simulink model "GPCA_CONFIGNoActions"  (Simulink 9.0)
settings: Solver=FixedStepDiscrete  StartTime=0.0  StopTime=10.0  RelTol=1e-3  EnableMultiTasking=on
settings Model: SuppressorTable=22 serialization::archive 11 0 6 0 0 0 0 0  Creator=bourbouh  LastModifiedBy=ktrinh
settings DataIOCC: SaveFormat=Dataset
settings DebuggingCC: UnderspecifiedInitializationDetection=Simplified  MergeDetectMultiDrivingBlocksExec=error
settings HardwareCC: ProdBitPerPointer=64  ProdBitPerSizeT=64  ProdBitPerPtrDiffT=64  ProdLargestAtomicFloat=Float  ProdIntDivRoundTo=Zero  ProdEndianess=LittleEndian  ProdWordSize=64  ProdHWDeviceType=Intel->x86-64 (Windows64)
settings ModelReferenceCC: PropagateSignalLabelsOutOfModel=on
settings GRTTargetCC: GeneratePreprocessorConditionals=Disable all

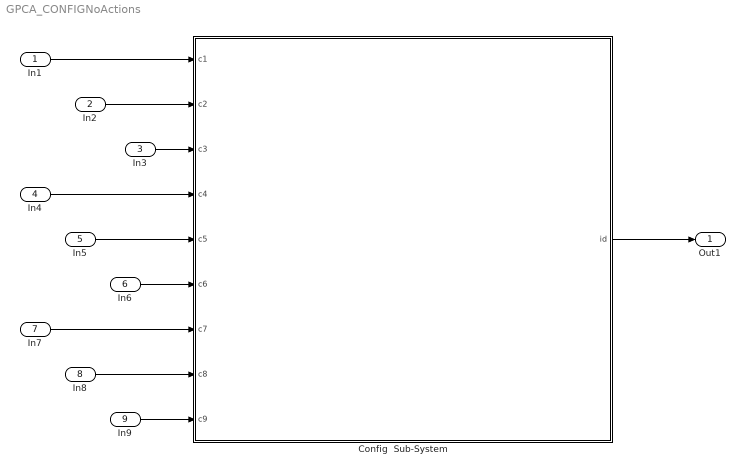
== system GPCA_CONFIGNoActions ==
  In1 : Inport  OutDataTypeStr=boolean
  In2 : Inport  Port=2  OutDataTypeStr=boolean
  In3 : Inport  Port=3  OutDataTypeStr=boolean
  In4 : Inport  Port=4  OutDataTypeStr=boolean
  In5 : Inport  Port=5  OutDataTypeStr=boolean
  In6 : Inport  Port=6  OutDataTypeStr=boolean
  In7 : Inport  Port=7  OutDataTypeStr=boolean
  In8 : Inport  Port=8  OutDataTypeStr=boolean
  In9 : Inport  Port=9  OutDataTypeStr=boolean
  Config  Sub-System : Stateflow chart  TreatAsAtomicUnit=on
  Out1 : Outport
  wires:
  Config  Sub-System/1(id) -> Out1/1
  In1/1 -> Config  Sub-System/1(c1)
  In9/1 -> Config  Sub-System/9(c9)
  In8/1 -> Config  Sub-System/8(c8)
  In7/1 -> Config  Sub-System/7(c7)
  In6/1 -> Config  Sub-System/6(c6)
  In5/1 -> Config  Sub-System/5(c5)
  In4/1 -> Config  Sub-System/4(c4)
  In3/1 -> Config  Sub-System/3(c3)
  In2/1 -> Config  Sub-System/2(c2)

== stateflow chart Config  Sub-System ==
  state Configuration
    en: id=2
    state Prescription_Config
      entry: id=22;
      state Patient_Drug_info
        entry: id=221;
        state GetParam
          entry: id = 222;
        state DisplayParam
          entry: id=222;
        state GetDrugSafeValues
          entry:id =224;
        state DisplayErrorMessage
          entry: id=223
        state ValidateParam
          entry: id=225;
        DisplayParam -> GetParam [order 1] : [ c7]
        (default) -> DisplayParam
        DisplayParam -> ValidateParam [order 2] : [ c6]
        DisplayErrorMessage -> DisplayParam
        GetParam -> GetDrugSafeValues : [c6]
        GetDrugSafeValues -> DisplayErrorMessage [order 2] : [c3]
        ValidateParam -> DisplayErrorMessage [order 1] : [c5]
        GetDrugSafeValues -> ValidateParam [order 1] : [c4]
      state SelectType
        entry: id = 23;
      state Infusion_info
        entry: id = 411;
        state GetInfusionParam
          entry: id=413;
        state RequestInfusionParam
          entry :id = 412;
        state ValidateInfusionParam
          entry: id = 414;
        RequestInfusionParam -> GetInfusionParam [order 1] : [ c4]
        (default) -> RequestInfusionParam
        ValidateInfusionParam -> RequestInfusionParam [order 1] : [c3]
        RequestInfusionParam -> ValidateInfusionParam [order 2] : [c2]
        GetInfusionParam -> ValidateInfusionParam : [ c5]
      state ConfirmInfusionInitation
        entry:id = 24;
      (default) -> SelectType
      SelectType -> (junction 23) : [c8]
      (junction 23) -> Patient_Drug_info [order 2] : [c1]
      (junction 23) -> Infusion_info [order 1] : [c9]
      Infusion_info -> Patient_Drug_info : [ c2]
      ValidateParam -> Infusion_info [order 2] : [c3]
      ValidateInfusionParam -> ConfirmInfusionInitation [order 2] : [c6]
    state MAIN
      entry: id = 21;
    (default) -> MAIN
    MAIN -> Prescription_Config : [c4]
    Prescription_Config -> MAIN : [c5]
    ConfirmInfusionInitation -> MAIN : [c6]
  state NOT_ON
    en: id=1
  (default) -> Configuration [order 1] : [c3]
  (default) -> NOT_ON [order 2]
  NOT_ON -> Configuration : [c1]
  Configuration -> NOT_ON : [c2]
  data: c1 input boolean; c2 input boolean; c3 input boolean; c4 input boolean; c5 input boolean; c6 input boolean; c7 input boolean; c8 input boolean; c9 input boolean; id output double
